simulink model "ComunicacionSerial"  (R2022b)
settings: Solver=VariableStepAuto  StartTime=0.0  StopTime=10.0  RelTol=1e-3
libraries: arduinolib x1
settings Model: Creator=David  LastModifiedBy=David

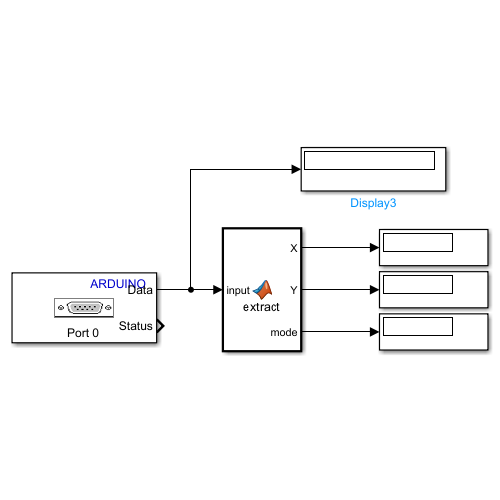
[thumbnail: Simulink's stored preview of the top-level diagram]
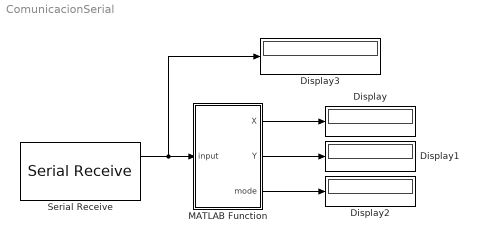
== system ComunicacionSerial ==
  Display{,1..3} (4 alike) : Display
  MATLAB Function : MATLAB Function  TreatAsAtomicUnit=on
  Serial Receive : arduinolib/Serial Receive  isARMArch=off  portNumber=0  DataType=int8  Datalength=30  SampleTime=-1  showOutStatus=on  blockPlatform=arduino
  wires:
  Serial Receive/1 -> Display3/1, MATLAB Function/1(input)
  MATLAB Function/3(mode) -> Display2/1
  MATLAB Function/2(Y) -> Display1/1
  MATLAB Function/1(X) -> Display/1

== matlab function ComunicacionSerial/MATLAB Function ==
  data: input input; X output; Y output; mode output
function [X,Y,mode] = extract(input)
% Decodificamos el objeto JSON
JSONdata = jsondecode(input);

X = JSONdata.X;
Y = JSONdata.Y;
mode = JSONdata.Button;

end
